simulink model "Main"  (R2023a)
settings: Solver=FixedStepAuto  StartTime=0.0  StopTime=1000  FixedStep=0.025  MaxStep=0.025  RelTol=1e-3
PreLoadFcn:
  | load WP.mat
undefined symbols (not defined in the file): TugStart, WP
libraries: simulink x2
settings Model: Creator=henni  LastModifiedBy=rkr021
settings OptimizationCC: ReuseModelBlockBuffer=off
settings DebuggingCC: UnconnectedInputMsg=warning  UnconnectedOutputMsg=warning  UnconnectedLineMsg=warning  UnderSpecifiedDimensionMsg=warning
settings ModelReferenceCC: EnableRefExpFcnMdlSchedulingChecks=on
settings RTWCC: DLArmComputeVersion=19.05
settings ConfigComp: DVTestSuiteOptimization=Auto  DVDetectOutOfBounds=on  DVModelReferenceHarness=on  DVHarnessSource=Signal Editor

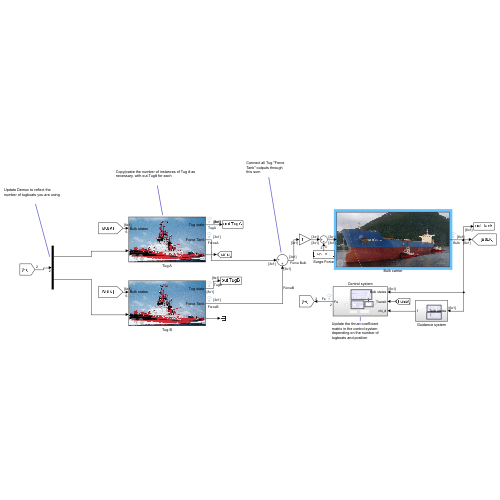
[thumbnail: Simulink's stored preview of the top-level diagram]
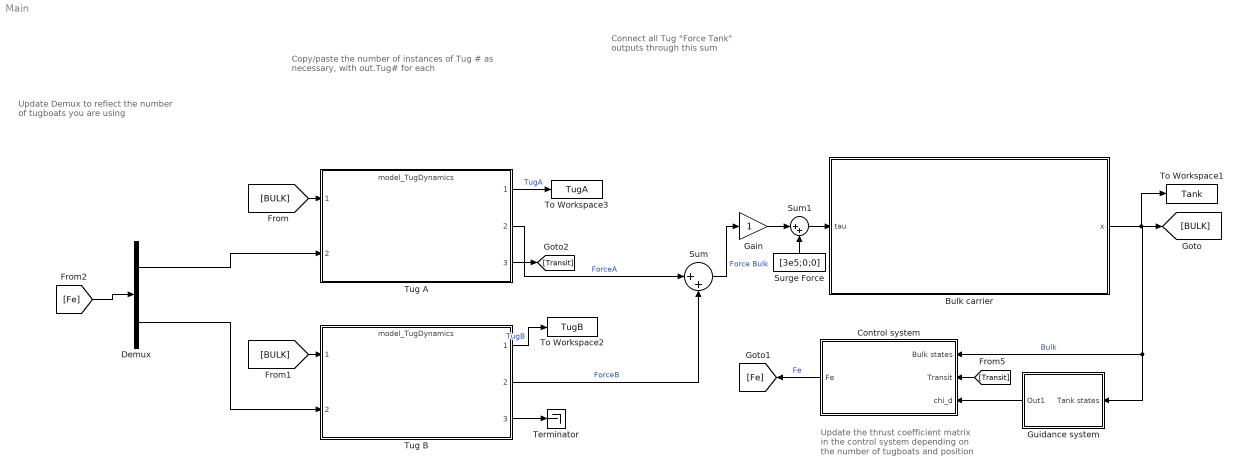
== system Main ==
  note: Update Demux to reflect the number of tugboats you are using
  note: Connect all Tug "Force Tank" outputs through this sum
  note: Copy/paste the number of instances of Tug # as necessary, with out.Tug# for each
  note: Update the thrust coefficient matrix in the control system depending on the number of tugboats and position
  Bulk carrier : Subsystem  mask{StartBulk=[0;0;deg2rad(90);0;0;deg2rad(0)]}
      mask prompts: StartBulk "Start position of bulk [x,y,psi,u,v,r]"
      mask Display: image('$imagefile'); % Use "Edit Image" on toolstrip to change.
  Control system : Subsystem
  Demux : Demux  Outputs=2
  Gain : Gain
  Guidance system : Subsystem
  Sum : Sum  Inputs=|++
  Sum1 : Sum  Inputs=|++
  Surge Force : Constant  Value=[3e5;0;0]
  Terminator : Terminator
  To Workspace1 : ToWorkspace  VariableName=Tank  SampleTime=-1
  To Workspace2 : ToWorkspace  VariableName=TugB  SampleTime=-1
  To Workspace3 : ToWorkspace  VariableName=TugA  SampleTime=-1
  Tug A : ModelReference  ModelNameDialog=model_TugDynamics.slx  UsingDefaultArgumentValue=0,0,0  SimulationMode=Normal  ModelReferenceVersion=3.1  StartTug=[40.5;80;deg2rad(180);0;0;deg2rad(0)]  Towline=60  Point=[80;-23]
  Tug B : ModelReference  ModelNameDialog=model_TugDynamics.slx  UsingDefaultArgumentValue=0,0,0  SimulationMode=Normal  ModelReferenceVersion=3.1  StartTug=[40.5;-80;deg2rad(180);0;0;deg2rad(0)]  Towline=60  Point=[-80;-23]
  wires:
  Tug A/1 -> To Workspace3/1  "TugA"
  Bulk carrier/1(x) -> Guidance system/1(Tank states), Control system/1(Bulk states), To Workspace1/1, [BULK]  "Bulk"
  Tug A/2 -> Sum/1  "ForceA"
  [BULK] -> Tug A/1
  [BULK] -> Tug B/1
  Tug B/2 -> Sum/2  "ForceB"
  Tug B/1 -> To Workspace2/1  "TugB"
  Sum1/1 -> Bulk carrier/1(tau)
  Surge Force/1 -> Sum1/2
  Demux/2 -> Tug B/2
  [Fe] -> Demux/1
  Tug B/3 -> Terminator/1
  Tug A/3 -> [Transit]
  Guidance system/1(Out1) -> Control system/3(chi_d)
  [Transit] -> Control system/2(Transit)
  Control system/1(Fe) -> [Fe]  "Fe"
  Demux/1 -> Tug A/2
  Gain/1 -> Sum1/1
  Sum/1 -> Gain/1  "Force Bulk"

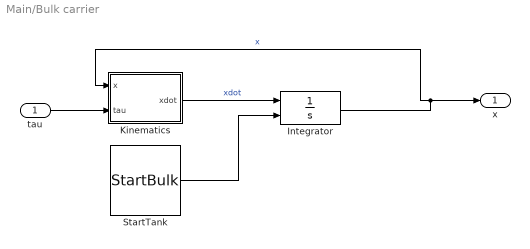
== system Main/Bulk carrier ==
  tau : Inport
  Integrator : Integrator  InitialConditionSource=external  InitialCondition=[0;0;0;0;0;0]
  "Kinematics " : MATLAB Function  TreatAsAtomicUnit=on
  StartTank : Constant  Value=StartBulk
  x : Outport
  wires:
  Integrator/1 -> x/1, "Kinematics "/1(x)  "x"
  "Kinematics "/1(xdot) -> Integrator/1  "xdot"
  StartTank/1 -> Integrator/2
  tau/1 -> "Kinematics "/2(tau)

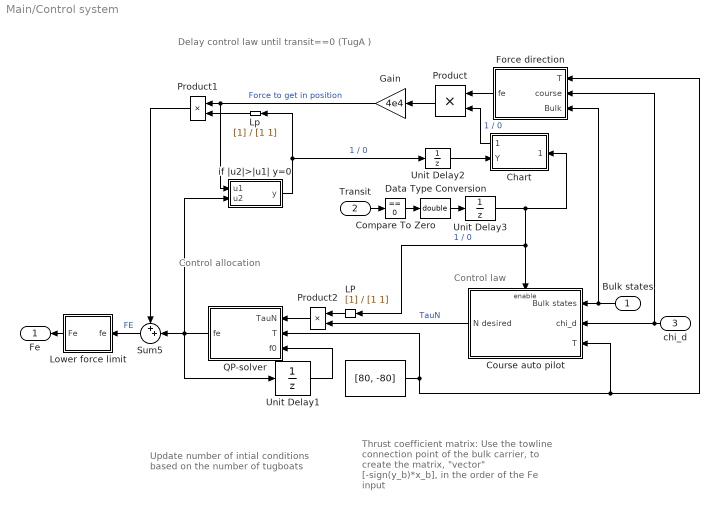
== system Main/Control system ==
  note: Update number of intial conditions based on the number of tugboats
  note: Delay control law until transit==0 (TugA )
  note: Thrust coefficient matrix:
      | Use the towline connection point of the bulk carrier, to create the matrix, "vector" [-sign(y_b)*x_b], in the order of the Fe input
  note: Control allocation
  note: Control law
  Bulk states : Inport
  Transit : Inport  Port=2
  chi_d : Inport  Port=3
  " " : Constant  Value=[80, -80]  VectorParams1D=off
  Chart : Stateflow chart  TreatAsAtomicUnit=on
      settings: PortSchema="{\"entries\":[{\"content\":{\"sides\":[{\"content\":{\"connectorIds\":[]},\"type\":\"ConnectorPlacement.EquallySpacedRectSide\",\"uuid\":\"eb5524b0-4aff-4dae-af04-54179d4fbde2\"},{\"content\":{\"connectorIds\":[],\"side\":\"RIGHT\"},\"type\":\"ConnectorPlacement.EquallySpacedRectSide\",\"uuid\":\"1a5e9ab8-0d12-48f5-9e34-ef9314eb5285\"},{\"content\":{\"connectorIds\":[\"In2\",\"Out1\"],\"side\":\"TOP\"},\"type\":\"ConnectorPlacement.EquallySpacedRectSide\",\"uuid\":\"2314afdb-540d-4892-a23a-3e1f75ede9b3\"},{\"content\":{\"connectorIds\":[\"In1\"],\"side\":\"BOTTOM\"},\"type\":\"ConnectorPlacement.EquallySpacedRectSide\",\"uuid\":\"2527712f-0a73-426f-9301-29e3ccd737f2\"}]},\"type\":\"ConnectorPlacement.EquallySpacedConnector\",\"uuid\":\"26fad560-b4c7-4ac4-99fb-aaadc92b0670\"}],\"packageUris\":[\"http://schema.mathworks.com/mf0/Connector/R2020b\"],\"version\":\"1.0\"}"
  Compare To Zero : simulink/Logic and Bit Operations/Compare To Zero  relop===  OutDataTypeStr=boolean
  Course auto pilot : Subsystem
  Data Type Conversion : DataTypeConversion  OutDataTypeStr=double  SaturateOnIntegerOverflow=off  RndMeth=Floor
  Force direction : MATLAB Function  TreatAsAtomicUnit=on
  Gain : Gain  Gain=4e4
  LP : TransferFcn  Denominator=[1 1]
  Lower force limit : MATLAB Function  TreatAsAtomicUnit=on
  Lp : TransferFcn  Denominator=[1 1]
  Product : Product
  Product1 : Product
  Product2 : Product
  QP-solver : MATLAB Function  TreatAsAtomicUnit=on
  Sum5 : Sum  Inputs=++|
  Unit Delay1 : UnitDelay  InitialCondition=zeros(2,1)  SampleTime=-1  HasFrameUpgradeWarning=on
  Unit Delay2 : UnitDelay  SampleTime=-1  HasFrameUpgradeWarning=on
  Unit Delay3 : UnitDelay  SampleTime=-1  HasFrameUpgradeWarning=on
  if |u2|>|u1| y=0 : MATLAB Function  TreatAsAtomicUnit=on
  Fe : Outport
  wires:
  Gain/1 -> if |u2|>|u1| y=0/1(u1), Product1/1  "Force to get in position"
  " "/1 -> Force direction/1(T), Course auto pilot/3(T), QP-solver/2(T)
  Unit Delay3/1 -> LP/1, Course auto pilot/Enable, Chart/1(Active)  "1 / 0"
  Lp/1 -> Product1/2
  Force direction/1(fe) -> Product/1
  QP-solver/1(fe) -> Unit Delay1/1, Sum5/2, if |u2|>|u1| y=0/2(u2)
  if |u2|>|u1| y=0/1(y) -> Lp/1, Unit Delay2/1  "1 / 0"
  Chart/1(State) -> Product/2  "1 / 0"
  Product2/1 -> QP-solver/1(TauN)
  Bulk states/1 -> Force direction/3(Bulk), Course auto pilot/1(Bulk states)
  Compare To Zero/1 -> Data Type Conversion/1
  Product1/1 -> Sum5/1
  Data Type Conversion/1 -> Unit Delay3/1
  Transit/1 -> Compare To Zero/1
  chi_d/1 -> Course auto pilot/2(chi_d), Force direction/2(course)
  LP/1 -> Product2/1
  Unit Delay2/1 -> Chart/2(Y)
  Unit Delay1/1 -> QP-solver/3(f0)
  Course auto pilot/1(N desired) -> Product2/2  "TauN"
  Sum5/1 -> Lower force limit/1(fe)  "FE"
  Lower force limit/1(Fe) -> Fe/1
  Product/1 -> Gain/1

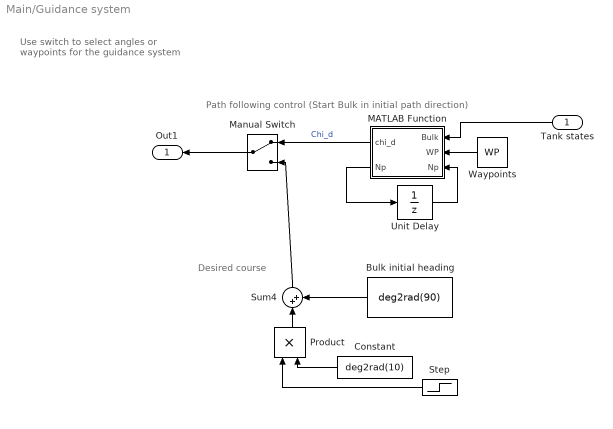
== system Main/Guidance system ==
  note: Use switch to select angles or waypoints for the guidance system
  note: Desired course
  note: Path following control (Start Bulk in initial path direction)
  Tank states : Inport
  Bulk initial heading : Constant  Value=deg2rad(90)
  Constant : Constant  Value=deg2rad(10)
  MATLAB Function : MATLAB Function  TreatAsAtomicUnit=on
  Manual Switch : ManualSwitch
  Product : Product
  Step : Step  Time=500  Before=1  After=-1  SampleTime=0
  Sum4 : Sum  Inputs=|++
  Unit Delay : UnitDelay  InitialCondition=1  SampleTime=-1  HasFrameUpgradeWarning=on
  Waypoints : Constant  Value=WP  VectorParams1D=off
  Out1 : Outport
  wires:
  Waypoints/1 -> MATLAB Function/2(WP)
  Constant/1 -> Product/2
  Step/1 -> Product/1
  Unit Delay/1 -> MATLAB Function/3("Np ")
  Bulk initial heading/1 -> Sum4/2
  Product/1 -> Sum4/1
  Tank states/1 -> MATLAB Function/1(Bulk)
  MATLAB Function/1(chi_d) -> Manual Switch/1  "Chi_d"
  MATLAB Function/2(Np) -> Unit Delay/1
  Sum4/1 -> Manual Switch/2
  Manual Switch/1 -> Out1/1

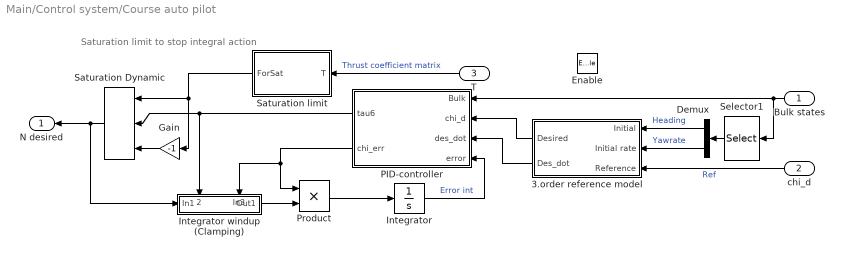
== system Main/Control system/Course auto pilot ==
  note: Saturation limit to stop integral action
  Bulk states : Inport
  chi_d : Inport  Port=2
  T : Inport  Port=3
  Enable : EnablePort  StatesWhenEnabling=reset
  3.order reference model : Subsystem  mask{wn=0.02, zeta=1.5, sat_rd=deg2rad(0.15), sat_ad=deg2rad(0.002)}
      mask prompts: wn "Natural frequency:"; zeta "Relative damping:"; sat_rd "Saturation eta_d_dot:"; sat_ad "Saturation eta_d_Ddot:"
  Demux : Demux  Outputs=2
  Gain : Gain  Gain=-1
  Integrator : Integrator
  Integrator windup (Clamping) : Subsystem
      settings: PortSchema="{\"entries\":[{\"content\":{\"sides\":[{\"content\":{\"connectorIds\":[\"In1\"]},\"type\":\"ConnectorPlacement.EquallySpacedRectSide\",\"uuid\":\"5f6056ac-e27d-4265-b11b-e690ab01c032\"},{\"content\":{\"connectorIds\":[\"Out1\"],\"side\":\"RIGHT\"},\"type\":\"ConnectorPlacement.EquallySpacedRectSide\",\"uuid\":\"89884b76-4881-4ea6-aa7d-0afa5529496d\"},{\"content\":{\"connectorIds\":[\"In2\",\"In3\"],\"side\":\"TOP\"},\"type\":\"ConnectorPlacement.EquallySpacedRectSide\",\"uuid\":\"1da8c3fb-635e-46e0-b348-e329ca47a2ec\"}]},\"type\":\"ConnectorPlacement.EquallySpacedConnector\",\"uuid\":\"5e14f300-2fc5-4e6c-905e-32da7616b803\"}],\"packageUris\":[\"http://schema.mathworks.com/mf0/Connector/R2020b\"],\"version\":\"1.0\"}"
  PID-controller : MATLAB Function  TreatAsAtomicUnit=on  SystemSampleTime=1
  Product : Product  OutDataTypeStr=Inherit: Same as first input
  Saturation Dynamic : simulink/Discontinuities/Saturation Dynamic  OutMin=[]  OutMax=[]  OutDataTypeStr=Inherit: Same as second input  OutDataType=fixdt(1, 16)  OutScaling=2^-10  DoSatur=off
  Saturation limit : MATLAB Function  TreatAsAtomicUnit=on
  Selector1 : Selector  InputPortWidth=6  IndexOptions=Index vector (dialog)  Indices=[3,6]  OutputSizes=1
  N desired : Outport
  wires:
  Integrator/1 -> PID-controller/4(error)  "Error int"
  chi_d/1 -> 3.order reference model/3(Reference)  "Ref"
  Demux/1 -> 3.order reference model/1(Initial)  "Heading"
  3.order reference model/1(Desired) -> PID-controller/2(chi_d)
  Demux/2 -> 3.order reference model/2(Initial rate)  "Yawrate"
  Saturation Dynamic/1 -> N desired/1, Integrator windup (Clamping)/1(In1)
  Product/1 -> Integrator/1
  Selector1/1 -> Demux/1
  3.order reference model/2(Des_dot) -> PID-controller/3(des_dot)
  Bulk states/1 -> PID-controller/1(Bulk), Selector1/1
  PID-controller/2(chi_err) -> Integrator windup (Clamping)/3(In3), Product/1
  Saturation limit/1(ForSat) -> Gain/1, Saturation Dynamic/1
  Integrator windup (Clamping)/1(Out1) -> Product/2
  Gain/1 -> Saturation Dynamic/3
  PID-controller/1(tau6) -> Saturation Dynamic/2, Integrator windup (Clamping)/2(Desired Yaw moment)
  T/1 -> Saturation limit/1(T)  "Thrust coefficient matrix"

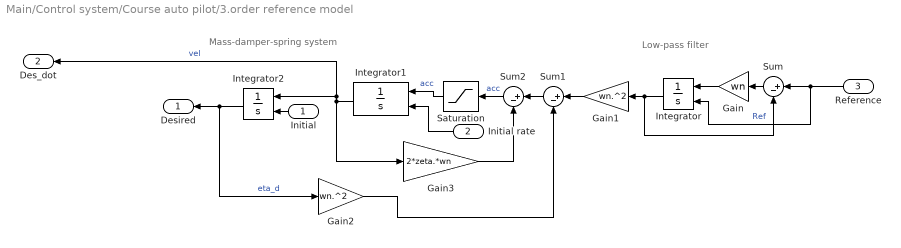
== system Main/Control system/Course auto pilot/3.order reference model ==
  note: Low-pass filter
  note: Mass-damper-spring system
  Initial : Inport
  Initial rate : Inport  Port=2
  Reference : Inport  Port=3
  Gain : Gain  Gain=wn
  Gain1 : Gain  Gain=wn.^2
  Gain2 : Gain  Gain=wn.^2
  Gain3 : Gain  Gain=2*zeta.*wn
  Integrator : Integrator  InitialConditionSource=external  InitialCondition=TugStart
  Integrator1 : Integrator  InitialConditionSource=external  LimitOutput=on  UpperSaturationLimit=sat_rd  LowerSaturationLimit=-sat_rd
  Integrator2 : Integrator  InitialConditionSource=external  InitialCondition=TugStart
  Saturation : Saturate  UpperLimit=sat_ad  LowerLimit=-sat_ad
  Sum : Sum  Inputs=|+-
  Sum1 : Sum  Inputs=|+-
  Sum2 : Sum  Inputs=|+-
  Desired : Outport
  Des_dot : Outport  Port=2
  wires:
  Gain/1 -> Integrator/1
  Integrator/1 -> Gain1/1, Sum/2
  Sum/1 -> Gain/1
  Gain1/1 -> Sum1/1
  Sum2/1 -> Saturation/1  "acc"
  Integrator1/1 -> Des_dot/1, Integrator2/1, Gain3/1  "vel"
  Integrator2/1 -> Desired/1, Gain2/1  "eta_d"
  Gain2/1 -> Sum1/2
  Initial/1 -> Integrator2/2
  Saturation/1 -> Integrator1/1  "acc"
  Reference/1 -> Integrator/2, Sum/1  "Ref"
  Initial rate/1 -> Integrator1/2
  Sum1/1 -> Sum2/1
  Gain3/1 -> Sum2/2

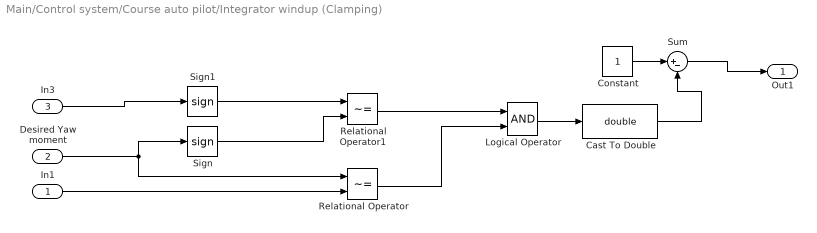
== system Main/Control system/Course auto pilot/Integrator windup (Clamping) ==
  In1 : Inport
  Desired Yaw moment : Inport  Port=2
  In3 : Inport  Port=3
  Cast To Double : DataTypeConversion  OutDataTypeStr=double  SaturateOnIntegerOverflow=off  RndMeth=Floor
  Constant : Constant
  Logical Operator : Logic  AllPortsSameDT=off  OutDataTypeStr=boolean
  Relational Operator : RelationalOperator  Operator=~=  OutDataTypeStr=boolean  RndMeth=Simplest  InputSameDT=off
  Relational Operator1 : RelationalOperator  Operator=~=  OutDataTypeStr=boolean  RndMeth=Simplest  InputSameDT=off
  Sign : Signum
  Sign1 : Signum
  Sum : Sum  Inputs=|+-
  Out1 : Outport
  wires:
  Relational Operator1/1 -> Logical Operator/1
  Sign/1 -> Relational Operator1/2
  Desired Yaw moment/1 -> Sign/1, Relational Operator/1
  In3/1 -> Sign1/1
  Sign1/1 -> Relational Operator1/1
  Relational Operator/1 -> Logical Operator/2
  In1/1 -> Relational Operator/2
  Logical Operator/1 -> Cast To Double/1
  Cast To Double/1 -> Sum/2
  Constant/1 -> Sum/1
  Sum/1 -> Out1/1

== matlab function Main/Control system/Force direction ==
  data: T input; course input; Bulk input; fe output
function fe = fcn(T, course,Bulk)
 
psiTilde = ssa(Bulk(3)-course);

if abs(psiTilde)<=deg2rad(0.1)
    fe=zeros(1,length(T));
else
    if psiTilde<0
        fe = sign(T);
    elseif psiTilde>0
        fe =-sign(T);
    else
        fe=zeros(1,length(T));
    end
end

== matlab function Main/Control system/Course auto pilot/PID-controller ==
  data: Bulk input; tau6 output; chi_d input; des_dot input; error input; chi_err output
function [tau6,chi_err]  = CoursePID(Bulk, chi_d,des_dot, error)
psi=Bulk(3);
% u = Bulk(4); v=Bulk(5); 
r=Bulk(6);
wb      = 0.064;%64*5;   % Control bandwidth
zeta    = 1;        % Relative damping
% psi   = heading angle
% nu    = linear and angular velocity vector [u,v,r]
% chi_d = Desired course angle
% error = Integrated error in the course angle


% if abs(v)>=0.01
% beta_c = asin(v/((u^2+v^2)^(0.5))); 
% else
   beta_c=0;  
% end
chi     = psi+beta_c; 
chi_dot = r-des_dot;        %Setting the crab angle to be constant error  
chi_err = ssa(chi-chi_d); 

[Kp,Kd,Ki] = CourseAutoP(wb,zeta);

tau6 = - Kp*chi_err -Kd*chi_dot -Ki*error;

== matlab function Main/Control system/QP-solver ==
  data: TauN input; T input; fe output; f0 input
function fe = fcn(TauN,T,f0)
dMax = 50e4/10*0.025;
f_max=ones(length(T),1)*50e4;
f_min=-f_max;
fe = QPsolver_Bulk(TauN,T,f0,dMax,f_max,f_min);

== matlab function Main/Guidance system/MATLAB Function ==
  data: Bulk input; WP input; Np input; chi_d output; Np output
function [chi_d,Np]= fcn(Bulk,WP,Np)
Xp      = WP(1,:); 
Yp      = WP(2,:); 

xp  = Xp(Np:Np+1);
yp  = Yp(Np:Np+1);

% cross-track error expressed in NED
Nab = 50;
pi_p = atan2(yp(2)-yp(1), xp(2)-xp(1));
 [x_p, y_p, y_e] = crosstrack(xp(2), yp(2), xp(1), yp(1), Bulk(1), Bulk(2));
  x_p   = x_p+Nab*cos(pi_p);
  y_p   = y_p+Nab*sin(pi_p); 


  Kp= 1/Nab; % 1/lookahead distance, 
    chi_d =  pi_p-atan(Kp*y_e);

  distance = ((xp(2)-x_p)^2+(yp(2)-y_p)^2)^(1/2);

  
Max = length(Xp)-1;
  if distance<1 && Np<Max
      Np=Np+1;
  end
% % % Book p.356

== matlab function Main/Control system/Course auto pilot/Saturation limit ==
  data: T input; ForSat output
function ForSat = saturationLim(T)
n = length(T);          % Number of tugboats
Dist = mean(abs(T));    % Mean distance from CO
ForSat = n*Dist*50e4;   % Saturation limit to cancel out integral action

== matlab function Main/Bulk carrier/Kinematics  ==
  data: x input; xdot output; tau input
function xdot = fcn(x,tau)
% x = [eta;nu] = [xn;yn;psi;u;v;r]; 

[etaDot,nuDot] = TankerDynamics(x,tau);

xdot = [etaDot;nuDot];

== stateflow chart Main/Control system/Chart ==
  (default) -> (junction 24)
  (junction 24) -> (junction 25) [order 1] : [[Y==0 && Active==1]]
  (junction 24) -> (junction 26) [order 2] : {State=1;}
  (junction 25) -> (junction 27) : {State=0;}
  (junction 27) -> (junction 26)
  (junction 26) -> (junction 28)
  data: Active input; Y input; State output

== matlab function Main/Control system/Lower force limit ==
  data: fe input; Fe output
function Fe = fcn(fe)


Low  = abs(fe)<=8e3;
fe(Low)=0;
Fe=fe;

== matlab function Main/Control system/if |u2|>|u1| y=0 ==
  data: u1 input; y output; u2 input
function y = fcn(u1, u2)



if abs(u2(1))>=abs(u1(1))
    y=0;
else
    y=1;
end
